simulink library "LIB_Warning"  (R2018b)
settings: Solver=VariableStepAuto  StartTime=0.0  StopTime=10.0  RelTol=1e-3
undefined symbols (not defined in the file or in its folder): eRespiratorStates, eSupervisorStates, rDecWarning, rIncpEndError, rIncpMinError, rIncpPlateauError, tBatteryErrorConfirmationDelay, tTBlowerMotorErrorConfirmationDelay
libraries: simulink x15, simulink_extras x3
settings Model: Creator=BRAUL  LastModifiedBy=BRAUL

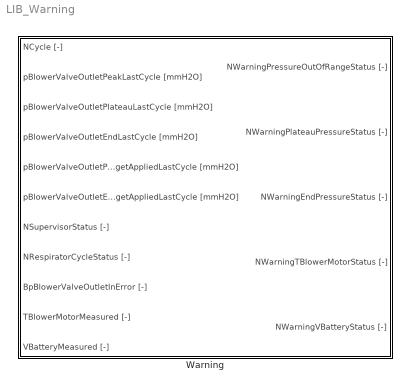
== system LIB_Warning ==
  Warning : Subsystem
      settings: AttributesFormatString=%<ReferenceBlock>

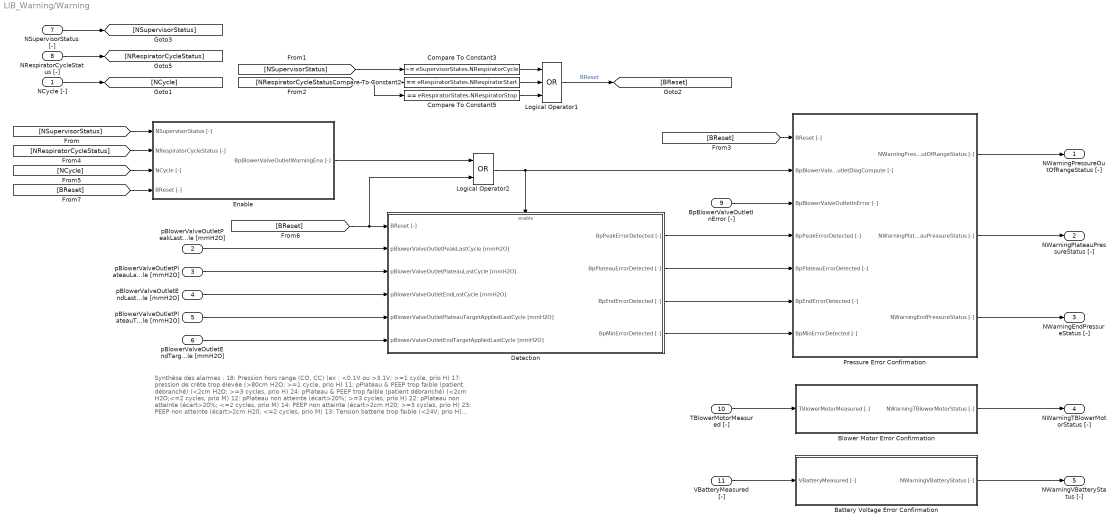
== system LIB_Warning/Warning ==
  note: Synthèse des alarmes :
      |
      | 18: Pression hors range (CO, CC) (ex : <0.1V ou >3.1V; >=1 cycle, prio H)
      | 17: pression de crête trop élevée (>80cm H2O; >=1 cycle, prio H)
      | 11: pPlateau & PEEP trop faible (patient débranché) (<2cm H2O; >=3 cycles, prio H)
      | 24: pPlateau & PEEP trop faible (patient débranché) (<2cm H2O;<=2 cycles, prio M)
      |
      | 12: pPlateau non atteinte (écart>20%; >=3 cycles, prio H)
      | 22: pPlateau non atteinte (écart>20%; <=2 cycles, prio M)
      |
      | 14: PEEP non atteinte (écart>2cm H20; >=3 cycles, prio H)
      | 23: PEEP non atteinte (écart>2cm H20; <=2 cycles, prio M)
      |
      | 13: Tension batterie trop faible (<24V; prio H)
      | 21: Tension batterie faible (<24.6V; prio M)
      | 31: Tension alimentation faible ( <=> secteur débranché)(<27V; prio L)
      |
      | 15: T moteur blower trop élevée (tempé>80°C; prio H)
  NCycle [-] : Inport
  pBlowerValveOutletPeakLastCycle [mmH2O] : Inport  Port=2
  pBlowerValveOutletPlateauLastCycle [mmH2O] : Inport  Port=3
  pBlowerValveOutletEndLastCycle [mmH2O] : Inport  Port=4
  pBlowerValveOutletPlateauTargetAppliedLastCycle [mmH2O] : Inport  Port=5
  pBlowerValveOutletEndTargetAppliedLastCycle [mmH2O] : Inport  Port=6
  NSupervisorStatus [-] : Inport  Port=7
  NRespiratorCycleStatus [-] : Inport  Port=8
  BpBlowerValveOutletInError [-] : Inport  Port=9
  TBlowerMotorMeasured [-] : Inport  Port=10
  VBatteryMeasured [-] : Inport  Port=11
  Battery Voltage Error Confirmation : Subsystem
  Blower Motor Error Confirmation : Subsystem
  Compare To Constant2 : simulink/Logic and Bit Operations/Compare To Constant  relop===  const=eRespiratorStates.NRespiratorStart  OutDataTypeStr=boolean
  Compare To Constant3 : simulink/Logic and Bit Operations/Compare To Constant  relop=~=  const=eSupervisorStates.NRespiratorCycle  OutDataTypeStr=boolean
  Compare To Constant5 : simulink/Logic and Bit Operations/Compare To Constant  relop===  const=eRespiratorStates.NRespiratorStop  OutDataTypeStr=boolean
  Detection : Subsystem
  Enable : Subsystem
  Logical Operator1 : Logic  Operator=OR  Inputs=3  AllPortsSameDT=off  OutDataTypeStr=boolean
  Logical Operator2 : Logic  Operator=OR  AllPortsSameDT=off  OutDataTypeStr=boolean
  Pressure Error Confirmation : Subsystem
  NWarningPressureOutOfRangeStatus [-] : Outport
  NWarningPlateauPressureStatus [-] : Outport  Port=2
  NWarningEndPressureStatus [-] : Outport  Port=3
  NWarningTBlowerMotorStatus [-] : Outport  Port=4
  NWarningVBatteryStatus [-] : Outport  Port=5
  wires:
  pBlowerValveOutletPlateauTargetAppliedLastCycle [mmH2O]/1 -> Detection/5(pBlowerValveOutletPlateauTargetAppliedLastCycle [mmH2O])
  pBlowerValveOutletEndLastCycle [mmH2O]/1 -> Detection/4(pBlowerValveOutletEndLastCycle [mmH2O])
  Battery Voltage Error Confirmation/1(NWarningVBatteryStatus [-]) -> NWarningVBatteryStatus [-]/1
  Blower Motor Error Confirmation/1(NWarningTBlowerMotorStatus [-]) -> NWarningTBlowerMotorStatus [-]/1
  Pressure Error Confirmation/3(NWarningEndPressureStatus [-]) -> NWarningEndPressureStatus [-]/1
  Pressure Error Confirmation/2(NWarningPlateauPressureStatus [-]) -> NWarningPlateauPressureStatus [-]/1
  Pressure Error Confirmation/1(NWarningPressureOutOfRangeStatus [-]) -> NWarningPressureOutOfRangeStatus [-]/1
  Enable/1(BpBlowerValveOutletWarningEna [-]) -> Logical Operator2/1
  [BReset] -> Logical Operator2/2, Detection/1(BReset [-])
  Logical Operator2/1 -> Detection/Enable, Pressure Error Confirmation/2(BpBlowerValveOutletDiagCompute [-])
  BpBlowerValveOutletInError [-]/1 -> Pressure Error Confirmation/3(BpBlowerValveOutletInError [-])
  TBlowerMotorMeasured [-]/1 -> Blower Motor Error Confirmation/1(TBlowerMotorMeasured [-])
  VBatteryMeasured [-]/1 -> Battery Voltage Error Confirmation/1(VBatteryMeasured [-])
  [BReset] -> Enable/4(BReset [-])
  [NCycle] -> Enable/3(NCycle [-])
  [NRespiratorCycleStatus] -> Enable/2(NRespiratorCycleStatus [-])
  pBlowerValveOutletEndTargetAppliedLastCycle [mmH2O]/1 -> Detection/6(pBlowerValveOutletEndTargetAppliedLastCycle [mmH2O])
  pBlowerValveOutletPlateauLastCycle [mmH2O]/1 -> Detection/3(pBlowerValveOutletPlateauLastCycle [mmH2O])
  pBlowerValveOutletPeakLastCycle [mmH2O]/1 -> Detection/2(pBlowerValveOutletPeakLastCycle [mmH2O])
  [BReset] -> Pressure Error Confirmation/1(BReset [-])
  [NSupervisorStatus] -> Enable/1(NSupervisorStatus [-])
  NCycle [-]/1 -> [NCycle]
  NRespiratorCycleStatus [-]/1 -> [NRespiratorCycleStatus]
  NSupervisorStatus [-]/1 -> [NSupervisorStatus]
  [NRespiratorCycleStatus] -> Compare To Constant5/1, Compare To Constant2/1
  Compare To Constant5/1 -> Logical Operator1/3
  [NSupervisorStatus] -> Compare To Constant3/1
  Compare To Constant3/1 -> Logical Operator1/1
  Logical Operator1/1 -> [BReset]  "BReset"
  Compare To Constant2/1 -> Logical Operator1/2
  Detection/4(BpMinErrorDetected [-]) -> Pressure Error Confirmation/7(BpMinErrorDetected [-])
  Detection/3(BpEndErrorDetected [-]) -> Pressure Error Confirmation/6(BpEndErrorDetected [-])
  Detection/2(BpPlateauErrorDetected [-]) -> Pressure Error Confirmation/5(BpPlateauErrorDetected [-])
  Detection/1(BpPeakErrorDetected [-]) -> Pressure Error Confirmation/4(BpPeakErrorDetected [-])

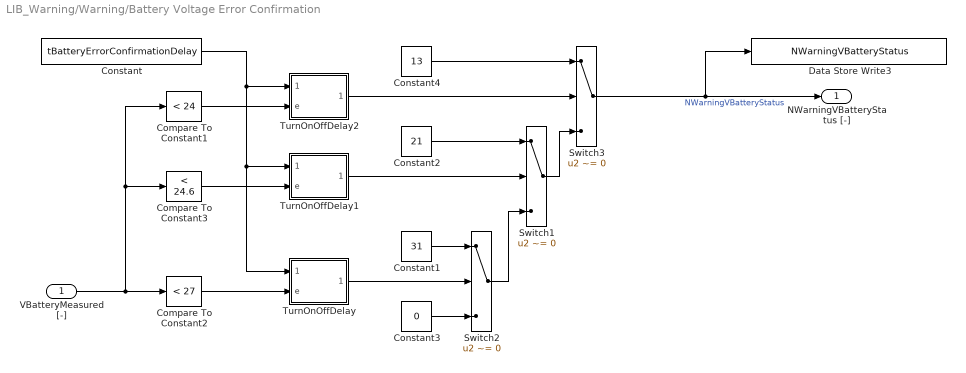
== system LIB_Warning/Warning/Battery Voltage Error Confirmation ==
  VBatteryMeasured [-] : Inport
  Compare To Constant1 : simulink/Logic and Bit Operations/Compare To Constant  relop=<  const=24  OutDataTypeStr=boolean
  Compare To Constant2 : simulink/Logic and Bit Operations/Compare To Constant  relop=<  const=27  OutDataTypeStr=boolean
  Compare To Constant3 : simulink/Logic and Bit Operations/Compare To Constant  relop=<  const=24.6  OutDataTypeStr=boolean
  Constant : Constant  Value=tBatteryErrorConfirmationDelay  OutDataTypeStr=single
  Constant1 : Constant  Value=31  OutDataTypeStr=uint8
  Constant2 : Constant  Value=21  OutDataTypeStr=uint8
  Constant3 : Constant  Value=0  OutDataTypeStr=uint8
  Constant4 : Constant  Value=13  OutDataTypeStr=uint8
  Data Store Write3 : DataStoreWrite  DataStoreName=NWarningVBatteryStatus
  Switch1 : Switch  Criteria=u2 ~= 0
      settings: AttributesFormatString=%<Criteria>
  Switch2 : Switch  Criteria=u2 ~= 0
      settings: AttributesFormatString=%<Criteria>
  Switch3 : Switch  Criteria=u2 ~= 0
      settings: AttributesFormatString=%<Criteria>
  TurnOnOffDelay : Subsystem  mask(TurnOn/OffDelay){DelayType=Turn On Delay, OutDataType=boolean}
      mask prompts: DelayType "Delay Type"; OutDataType "Out Data Type"
      mask help: Bloc de confirmation de montée/chute si e est/n'est plus vrai pendant une durée T (en secondes)
      mask init:
      | LogicBlocks=find_system(gcbh,'LookUnderMasks','all','FollowLinks','On','SearchDepth','1','BlockType','Logic');
      | DetectionBlock=find_system(gcbh,'LookUnderMasks','all','FollowLinks','On','SearchDepth','1','MaskType','DETECTIONFRONT');
      | if DelayType==1
      | set_param(LogicBlocks(1),'Operator','AND');
      | set_param(LogicBlocks(2),'Operator','AND');
      | set_param(DetectionBlock,'FrontType','Rising');
      | FrontIconY=[0.2 0.2 0.6 0.6];
      | else
      | set_param(LogicBlocks(1),'Operator','OR')
      | set_param(LogicBlocks(2),'Operator','NOT');
      | set_param(DetectionBlock,'FrontType','Falling');
      | FrontIconY=[0.6 0.6 0.2 0.2];
      | end
      | 
      | ConversionBlock=find_system(gcbh,'LookUnderMasks','all','FollowLinks','On','SearchDepth','1','BlockType','DataTypeConversion');
      | DataTypeOptionsStr=[{'Inherit: Inherit via back propagation'},{'double'},{'single'},{'int8'},{'uint8'},{'int16'},{'uint16'},{'int32'},{'uint32'},{'boolean'},{'fixdt(1,16)'},{'fixdt(1,16,0)'},{'fixdt(1,16,2^0,0)'},{'Enum: <class name>'},{'<data type expression>'}]
      | set_param(ConversionBlock,'OutDataTypeStr',DataTypeOptionsStr{OutDataType});
      settings: AttributesFormatString=%<StaticLinkStatus>
      mask TypeOptions DelayType: Turn On Delay | Turn Off Delay
      mask TypeOptions OutDataType: Inherit: Inherit via back propagation | double | single | int8 | uint8 | int16 | uint16 | int32 | uint32 | boolean | fixdt(1,16) | fixdt(1,16,0) | fixdt(1,16,2^0,0) | Enum: <class name> | <data type expression>
      mask Display:
      | plot([0.3 0.6 0.6 0.9], FrontIconY);
      | port_label('input',1,'T [s]')
      | port_label('input',2,'e')
      | text(0.4,0.4, 'T');
  TurnOnOffDelay1 : Subsystem  mask(TurnOn/OffDelay){DelayType=Turn On Delay, OutDataType=boolean}
      mask prompts: DelayType "Delay Type"; OutDataType "Out Data Type"
      mask help: Bloc de confirmation de montée/chute si e est/n'est plus vrai pendant une durée T (en secondes)
      mask init: same as LIB_Warning/Warning/Battery Voltage Error Confirmation/TurnOnOffDelay
      settings: AttributesFormatString=%<StaticLinkStatus>
      mask TypeOptions DelayType: Turn On Delay | Turn Off Delay
      mask TypeOptions OutDataType: Inherit: Inherit via back propagation | double | single | int8 | uint8 | int16 | uint16 | int32 | uint32 | boolean | fixdt(1,16) | fixdt(1,16,0) | fixdt(1,16,2^0,0) | Enum: <class name> | <data type expression>
      mask Display:
      | plot([0.3 0.6 0.6 0.9], FrontIconY);
      | port_label('input',1,'T [s]')
      | port_label('input',2,'e')
      | text(0.4,0.4, 'T');
  TurnOnOffDelay2 : Subsystem  mask(TurnOn/OffDelay){DelayType=Turn On Delay, OutDataType=boolean}
      mask prompts: DelayType "Delay Type"; OutDataType "Out Data Type"
      mask help: Bloc de confirmation de montée/chute si e est/n'est plus vrai pendant une durée T (en secondes)
      mask init: same as LIB_Warning/Warning/Battery Voltage Error Confirmation/TurnOnOffDelay
      settings: AttributesFormatString=%<StaticLinkStatus>
      mask TypeOptions DelayType: Turn On Delay | Turn Off Delay
      mask TypeOptions OutDataType: Inherit: Inherit via back propagation | double | single | int8 | uint8 | int16 | uint16 | int32 | uint32 | boolean | fixdt(1,16) | fixdt(1,16,0) | fixdt(1,16,2^0,0) | Enum: <class name> | <data type expression>
      mask Display:
      | plot([0.3 0.6 0.6 0.9], FrontIconY);
      | port_label('input',1,'T [s]')
      | port_label('input',2,'e')
      | text(0.4,0.4, 'T');
  NWarningVBatteryStatus [-] : Outport
  wires:
  Constant/1 -> TurnOnOffDelay2/1(DelayTime), TurnOnOffDelay1/1(DelayTime), TurnOnOffDelay/1(DelayTime)
  TurnOnOffDelay/1(Timer_end) -> Switch2/2
  TurnOnOffDelay1/1(Timer_end) -> Switch1/2
  TurnOnOffDelay2/1(Timer_end) -> Switch3/2
  Compare To Constant3/1 -> TurnOnOffDelay1/2(e)
  Compare To Constant1/1 -> TurnOnOffDelay2/2(e)
  Compare To Constant2/1 -> TurnOnOffDelay/2(e)
  Constant4/1 -> Switch3/1
  Constant2/1 -> Switch1/1
  Constant1/1 -> Switch2/1
  Constant3/1 -> Switch2/3
  Switch3/1 -> NWarningVBatteryStatus [-]/1, Data Store Write3/1  "NWarningVBatteryStatus"
  Switch1/1 -> Switch3/3
  Switch2/1 -> Switch1/3
  VBatteryMeasured [-]/1 -> Compare To Constant3/1, Compare To Constant1/1, Compare To Constant2/1

== system LIB_Warning/Warning/Blower Motor Error Confirmation ==
  TBlowerMotorMeasured [-] : Inport
  Compare To Constant2 : simulink/Logic and Bit Operations/Compare To Constant  relop=>  const=80  OutDataTypeStr=boolean
  Constant : Constant  Value=tTBlowerMotorErrorConfirmationDelay  OutDataTypeStr=single
  Constant1 : Constant  Value=15  OutDataTypeStr=uint8
  Constant3 : Constant  Value=0  OutDataTypeStr=uint8
  Data Store Write3 : DataStoreWrite  DataStoreName=NWarningTBlowerMotorStatus
  Switch2 : Switch  Criteria=u2 ~= 0
      settings: AttributesFormatString=%<Criteria>
  TurnOnOffDelay : Subsystem  mask(TurnOn/OffDelay){DelayType=Turn On Delay, OutDataType=boolean}
      mask prompts: DelayType "Delay Type"; OutDataType "Out Data Type"
      mask help: Bloc de confirmation de montée/chute si e est/n'est plus vrai pendant une durée T (en secondes)
      mask init: same as LIB_Warning/Warning/Battery Voltage Error Confirmation/TurnOnOffDelay
      settings: AttributesFormatString=%<StaticLinkStatus>
      mask TypeOptions DelayType: Turn On Delay | Turn Off Delay
      mask TypeOptions OutDataType: Inherit: Inherit via back propagation | double | single | int8 | uint8 | int16 | uint16 | int32 | uint32 | boolean | fixdt(1,16) | fixdt(1,16,0) | fixdt(1,16,2^0,0) | Enum: <class name> | <data type expression>
      mask Display:
      | plot([0.3 0.6 0.6 0.9], FrontIconY);
      | port_label('input',1,'T [s]')
      | port_label('input',2,'e')
      | text(0.4,0.4, 'T');
  NWarningTBlowerMotorStatus [-] : Outport
  wires:
  TBlowerMotorMeasured [-]/1 -> Compare To Constant2/1
  Switch2/1 -> NWarningTBlowerMotorStatus [-]/1, Data Store Write3/1  "NWarningTBlowerMotorStatus"
  Constant3/1 -> Switch2/3
  Constant1/1 -> Switch2/1
  Compare To Constant2/1 -> TurnOnOffDelay/2(e)
  TurnOnOffDelay/1(Timer_end) -> Switch2/2
  Constant/1 -> TurnOnOffDelay/1(DelayTime)

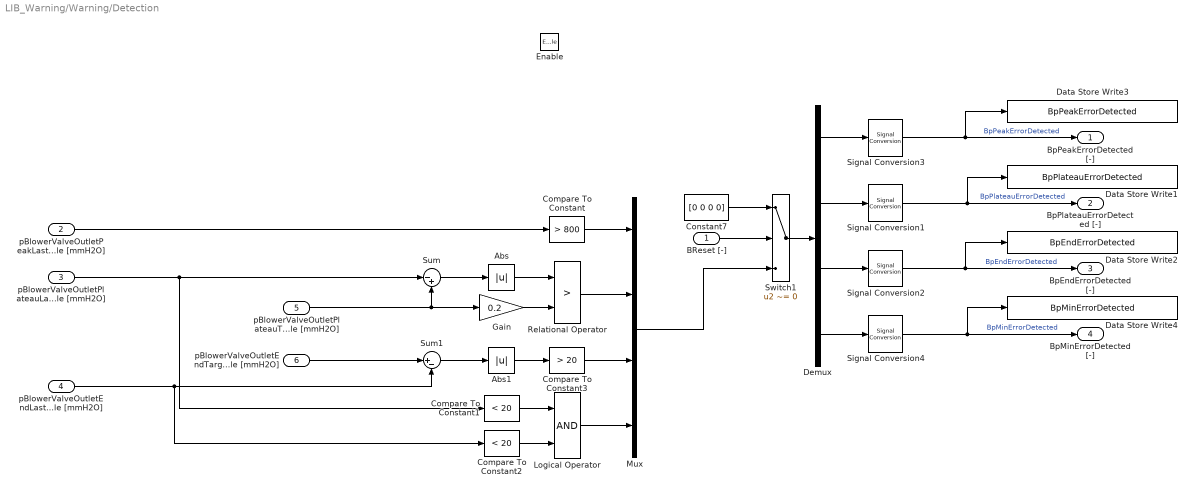
== system LIB_Warning/Warning/Detection ==
  BReset [-] : Inport
  pBlowerValveOutletPeakLastCycle [mmH2O] : Inport  Port=2
  pBlowerValveOutletPlateauLastCycle [mmH2O] : Inport  Port=3
  pBlowerValveOutletEndLastCycle [mmH2O] : Inport  Port=4
  pBlowerValveOutletPlateauTargetAppliedLastCycle [mmH2O] : Inport  Port=5
  pBlowerValveOutletEndTargetAppliedLastCycle [mmH2O] : Inport  Port=6
  Enable : EnablePort
  Abs : Abs
  Abs1 : Abs
  Compare To Constant : simulink/Logic and Bit Operations/Compare To Constant  relop=>  const=800  OutDataTypeStr=boolean
  Compare To Constant1 : simulink/Logic and Bit Operations/Compare To Constant  relop=<  const=20  OutDataTypeStr=boolean
  Compare To Constant2 : simulink/Logic and Bit Operations/Compare To Constant  relop=<  const=20  OutDataTypeStr=boolean
  Compare To Constant3 : simulink/Logic and Bit Operations/Compare To Constant  relop=>  const=20  OutDataTypeStr=boolean
  Constant7 : Constant  Value=[0 0 0 0]  OutDataTypeStr=boolean
  Data Store Write1 : DataStoreWrite  DataStoreName=BpPlateauErrorDetected
  Data Store Write2 : DataStoreWrite  DataStoreName=BpEndErrorDetected
  Data Store Write3 : DataStoreWrite  DataStoreName=BpPeakErrorDetected
  Data Store Write4 : DataStoreWrite  DataStoreName=BpMinErrorDetected
  Demux : Demux
  Gain : Gain  Gain=0.2
  Logical Operator : Logic  AllPortsSameDT=off  OutDataTypeStr=boolean
  Mux : Mux
  Relational Operator : RelationalOperator  Operator=>  OutDataTypeStr=boolean  RndMeth=Simplest
  Signal Conversion{1..4} (4 alike) : SignalConversion  OverrideOpt=off
  Sum : Sum  Inputs=|-+
  Sum1 : Sum  Inputs=|+-
  Switch1 : Switch  Criteria=u2 ~= 0
      settings: AttributesFormatString=%<Criteria>
  BpPeakErrorDetected [-] : Outport
  BpPlateauErrorDetected [-] : Outport  Port=2
  BpEndErrorDetected [-] : Outport  Port=3
  BpMinErrorDetected [-] : Outport  Port=4
  wires:
  Signal Conversion4/1 -> BpMinErrorDetected [-]/1, Data Store Write4/1  "BpMinErrorDetected"
  Signal Conversion2/1 -> BpEndErrorDetected [-]/1, Data Store Write2/1  "BpEndErrorDetected"
  Signal Conversion1/1 -> BpPlateauErrorDetected [-]/1, Data Store Write1/1  "BpPlateauErrorDetected"
  Signal Conversion3/1 -> BpPeakErrorDetected [-]/1, Data Store Write3/1  "BpPeakErrorDetected"
  Demux/4 -> Signal Conversion4/1
  Demux/3 -> Signal Conversion2/1
  Demux/2 -> Signal Conversion1/1
  Demux/1 -> Signal Conversion3/1
  Logical Operator/1 -> Mux/4
  Compare To Constant3/1 -> Mux/3
  Relational Operator/1 -> Mux/2
  Compare To Constant/1 -> Mux/1
  Mux/1 -> Switch1/3
  Switch1/1 -> Demux/1
  BReset [-]/1 -> Switch1/2
  Constant7/1 -> Switch1/1
  Abs1/1 -> Compare To Constant3/1
  Abs/1 -> Relational Operator/1
  Gain/1 -> Relational Operator/2
  pBlowerValveOutletPlateauTargetAppliedLastCycle [mmH2O]/1 -> Sum/2, Gain/1
  Compare To Constant1/1 -> Logical Operator/1
  Compare To Constant2/1 -> Logical Operator/2
  pBlowerValveOutletEndLastCycle [mmH2O]/1 -> Sum1/2, Compare To Constant2/1
  pBlowerValveOutletEndTargetAppliedLastCycle [mmH2O]/1 -> Sum1/1
  Sum1/1 -> Abs1/1
  pBlowerValveOutletPlateauLastCycle [mmH2O]/1 -> Compare To Constant1/1, Sum/1
  Sum/1 -> Abs/1
  pBlowerValveOutletPeakLastCycle [mmH2O]/1 -> Compare To Constant/1

== system LIB_Warning/Warning/Enable ==
  NSupervisorStatus [-] : Inport
  NRespiratorCycleStatus [-] : Inport  Port=2
  NCycle [-] : Inport  Port=3
  BReset [-] : Inport  Port=4
  Compare To Constant : simulink/Logic and Bit Operations/Compare To Constant  relop=>  const=1  OutDataTypeStr=boolean
  Compare To Constant1 : simulink/Logic and Bit Operations/Compare To Constant  relop===  const=eRespiratorStates.NRespiratorInInhalationPhase1  OutDataTypeStr=boolean
  Compare To Constant4 : simulink/Logic and Bit Operations/Compare To Constant  relop===  const=eSupervisorStates.NRespiratorCycle  OutDataTypeStr=boolean
  Constant6 : Constant  OutDataTypeStr=boolean
  Constant7 : Constant  Value=0  OutDataTypeStr=boolean
  Data Store Write3 : DataStoreWrite  DataStoreName=BpBlowerValveOutletWarningEna
  Detect Increase : simulink/Logic and Bit Operations/Detect Increase  vinit=0.0  OutDataTypeStr=boolean
  Logical Operator2 : Logic  Inputs=3  AllPortsSameDT=off  OutDataTypeStr=boolean
  Switch1 : Switch  Criteria=u2 ~= 0
      settings: AttributesFormatString=%<Criteria>
  Switch4 : Switch  Criteria=u2 ~= 0
      settings: AttributesFormatString=%<Criteria>
  Unit Delay1 : UnitDelay  SampleTime=-1
      settings: AttributesFormatString=%<InitialCondition>
  BpBlowerValveOutletWarningEna [-] : Outport
  wires:
  Compare To Constant/1 -> Switch4/2
  BReset [-]/1 -> Switch1/2
  NSupervisorStatus [-]/1 -> Compare To Constant4/1
  Detect Increase/1 -> Logical Operator2/2
  Constant7/1 -> Switch1/1
  NCycle [-]/1 -> Compare To Constant/1
  Unit Delay1/1 -> Switch4/3
  Switch1/1 -> Unit Delay1/1, Logical Operator2/3
  Constant6/1 -> Switch4/1
  NRespiratorCycleStatus [-]/1 -> Compare To Constant1/1
  Switch4/1 -> Switch1/3
  Logical Operator2/1 -> BpBlowerValveOutletWarningEna [-]/1, Data Store Write3/1  "BpBlowerValveOutletWarningEna"
  Compare To Constant1/1 -> Detect Increase/1
  Compare To Constant4/1 -> Logical Operator2/1

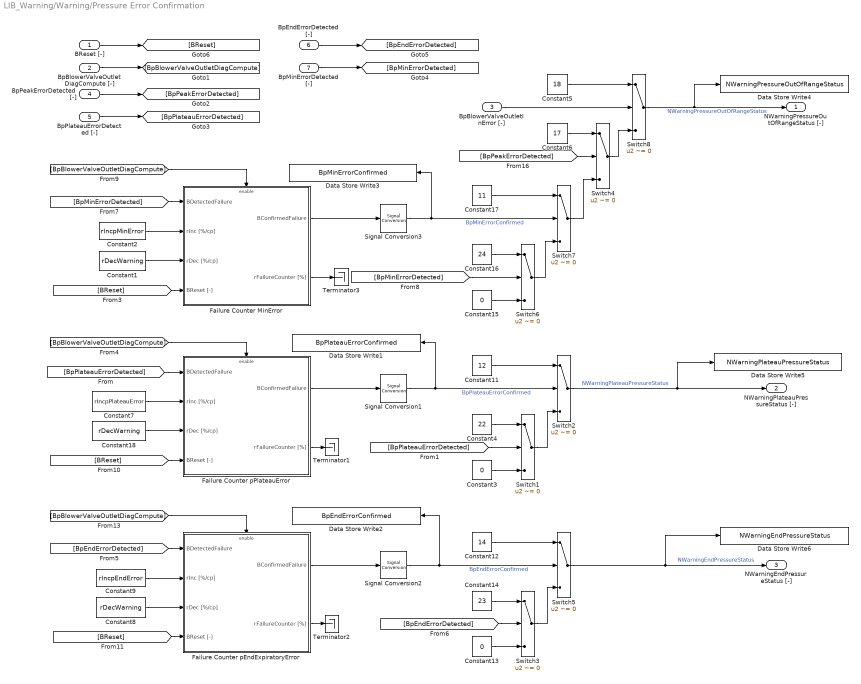
== system LIB_Warning/Warning/Pressure Error Confirmation ==
  BReset [-] : Inport
  BpBlowerValveOutletDiagCompute [-] : Inport  Port=2
  BpBlowerValveOutletInError [-] : Inport  Port=3
  BpPeakErrorDetected [-] : Inport  Port=4
  BpPlateauErrorDetected [-] : Inport  Port=5
  BpEndErrorDetected [-] : Inport  Port=6
  BpMinErrorDetected [-] : Inport  Port=7
  Constant1 : Constant  Value=rDecWarning  OutDataTypeStr=single
  Constant11 : Constant  Value=12  OutDataTypeStr=uint8
  Constant12 : Constant  Value=14  OutDataTypeStr=uint8
  Constant13 : Constant  Value=0  OutDataTypeStr=uint8
  Constant14 : Constant  Value=23  OutDataTypeStr=uint8
  Constant15 : Constant  Value=0  OutDataTypeStr=uint8
  Constant16 : Constant  Value=24  OutDataTypeStr=uint8
  Constant17 : Constant  Value=11  OutDataTypeStr=uint8
  Constant18 : Constant  Value=rDecWarning  OutDataTypeStr=single
  Constant2 : Constant  Value=rIncpMinError  OutDataTypeStr=single
  Constant3 : Constant  Value=0  OutDataTypeStr=uint8
  Constant4 : Constant  Value=22  OutDataTypeStr=uint8
  Constant5 : Constant  Value=18  OutDataTypeStr=uint8
  Constant6 : Constant  Value=17  OutDataTypeStr=uint8
  Constant7 : Constant  Value=rIncpPlateauError  OutDataTypeStr=single
  Constant8 : Constant  Value=rDecWarning  OutDataTypeStr=single
  Constant9 : Constant  Value=rIncpEndError  OutDataTypeStr=single
  Data Store Write1 : DataStoreWrite  DataStoreName=BpPlateauErrorConfirmed
  Data Store Write2 : DataStoreWrite  DataStoreName=BpEndErrorConfirmed
  Data Store Write3 : DataStoreWrite  DataStoreName=BpMinErrorConfirmed
  Data Store Write4 : DataStoreWrite  DataStoreName=NWarningPressureOutOfRangeStatus
  Data Store Write5 : DataStoreWrite  DataStoreName=NWarningPlateauPressureStatus
  Data Store Write6 : DataStoreWrite  DataStoreName=NWarningEndPressureStatus
  Failure Counter MinError : Subsystem  TreatAsAtomicUnit=on  mask(Failure Counter){temp=off, TSample=10, ena=on}
      mask prompts: temp "Is Temporal?"; TSample "Sample Time (ms)"; ena "Need to be Enable?"
      mask init:
      | %Find inputs to change name
      | rInc=find_system(gcbh,'LookUnderMasks','all','FollowLinks','on','RegExp','on','Name','rInc');
      | rDec=find_system(gcbh,'LookUnderMasks','all','FollowLinks','on','RegExp','on','Name','rDec');
      | rFail=find_system(gcbh,'LookUnderMasks','all','FollowLinks','on','RegExp','on','Name','rFail');
      | % Active enable
      | ena_block=find_system(gcbh,'LookUnderMasks','all','FollowLinks','on','Name','enable');
      | if ena && isempty(ena_block)  
      |     add_block('simulink/Ports & Subsystems/Enable',[gcb,'/enable'])
      | elseif not(ena) && not(isempty(ena_block))
      |     delete_block([gcb,'/enable']);
      | end
      | 
      | %Verify if Temporal or not
      | if temp
      |     set_param([gcb '/Sample'],'Value',mat2str(eval(TSample)))
      |     %sample=replace_block(gcbh,'Name','Sample','GDElib_functions/SampleTime','noprompt');
      |     %set_param(gcb,'DataType','single','TSample',mat2str(eval(TSample)/1000));
      |     set_param(rInc,'Name','rInc [%/ms]')
      |     set_param(rDec,'Name','rDec [%/ms]')
      |     set_param(rFail,'Name','rFailureCounter [%]')
      |     status=['Temporal \n' TSample ' ms'];
      | else
      |     set_param([gcb,'/Sample'],'Value','1');
      |     set_param(rInc,'Name','rInc [%/cp]')
      |     set_param(rDec,'Name','rDec [%/cp]')
      |     set_param(rFail,'Name','rFailureCounter [%]')
      |     status='Not Temporal';
      |     
      | end
      settings: AttributesFormatString=%<StaticLinkStatus>
      mask Callback temp:
      | maskedit_FailC=get_param(gcb,'temp');
      | vis_FailC = get_param(gcb, 'maskvisibilities');
      | vis_FailC{2} = maskedit_FailC;
      | set_param(gcb,'maskvisibilities',vis_FailC);
      | clear vis_FailC maskedit_FailC;
      mask TypeOptions TSample: 1 | 2 | 5 | 10 | 20 | 50 | 100 | 1000
      mask Display: disp(status)
  Failure Counter pEndExpiratoryError : Subsystem  TreatAsAtomicUnit=on  mask(Failure Counter){temp=off, TSample=10, ena=on}
      mask prompts: temp "Is Temporal?"; TSample "Sample Time (ms)"; ena "Need to be Enable?"
      mask init: same as LIB_Warning/Warning/Pressure Error Confirmation/Failure Counter MinError
      settings: AttributesFormatString=%<StaticLinkStatus>
      mask Callback temp:
      | maskedit_FailC=get_param(gcb,'temp');
      | vis_FailC = get_param(gcb, 'maskvisibilities');
      | vis_FailC{2} = maskedit_FailC;
      | set_param(gcb,'maskvisibilities',vis_FailC);
      | clear vis_FailC maskedit_FailC;
      mask TypeOptions TSample: 1 | 2 | 5 | 10 | 20 | 50 | 100 | 1000
      mask Display: disp(status)
  Failure Counter pPlateauError : Subsystem  TreatAsAtomicUnit=on  mask(Failure Counter){temp=off, TSample=10, ena=on}
      mask prompts: temp "Is Temporal?"; TSample "Sample Time (ms)"; ena "Need to be Enable?"
      mask init: same as LIB_Warning/Warning/Pressure Error Confirmation/Failure Counter MinError
      settings: AttributesFormatString=%<StaticLinkStatus>
      mask Callback temp:
      | maskedit_FailC=get_param(gcb,'temp');
      | vis_FailC = get_param(gcb, 'maskvisibilities');
      | vis_FailC{2} = maskedit_FailC;
      | set_param(gcb,'maskvisibilities',vis_FailC);
      | clear vis_FailC maskedit_FailC;
      mask TypeOptions TSample: 1 | 2 | 5 | 10 | 20 | 50 | 100 | 1000
      mask Display: disp(status)
  Signal Conversion1 : SignalConversion  OverrideOpt=off
  Signal Conversion2 : SignalConversion  OverrideOpt=off
  Signal Conversion3 : SignalConversion  OverrideOpt=off
  Switch{1..8} (8 alike) : Switch  Criteria=u2 ~= 0
      settings: AttributesFormatString=%<Criteria>
  Terminator1 : Terminator
  Terminator2 : Terminator
  Terminator3 : Terminator
  NWarningPressureOutOfRangeStatus [-] : Outport
  NWarningPlateauPressureStatus [-] : Outport  Port=2
  NWarningEndPressureStatus [-] : Outport  Port=3
  wires:
  [BpPeakErrorDetected] -> Switch4/2
  Constant5/1 -> Switch8/1
  BpBlowerValveOutletInError [-]/1 -> Switch8/2
  Switch4/1 -> Switch8/3
  Switch8/1 -> NWarningPressureOutOfRangeStatus [-]/1, Data Store Write4/1  "NWarningPressureOutOfRangeStatus"
  [BReset] -> Failure Counter pPlateauError/4(BReset [-])
  [BReset] -> Failure Counter pEndExpiratoryError/4(BReset [-])
  [BpBlowerValveOutletDiagCompute] -> Failure Counter pPlateauError/Enable
  [BpBlowerValveOutletDiagCompute] -> Failure Counter MinError/Enable
  [BReset] -> Failure Counter MinError/4(BReset [-])
  BReset [-]/1 -> [BReset]
  Switch5/1 -> NWarningEndPressureStatus [-]/1, Data Store Write6/1  "NWarningEndPressureStatus"
  Switch2/1 -> NWarningPlateauPressureStatus [-]/1, Data Store Write5/1  "NWarningPlateauPressureStatus"
  Switch7/1 -> Switch4/3
  Constant17/1 -> Switch7/1
  Constant16/1 -> Switch6/1
  Switch6/1 -> Switch7/3
  Signal Conversion3/1 -> Switch7/2, Data Store Write3/1  "BpMinErrorConfirmed"
  Failure Counter MinError/1(BConfirmedFailure) -> Signal Conversion3/1
  Failure Counter MinError/2(rFailureCounter [%]) -> Terminator3/1
  Constant15/1 -> Switch6/3
  [BpMinErrorDetected] -> Switch6/2
  [BpMinErrorDetected] -> Failure Counter MinError/1(BDetectedFailure)
  Failure Counter pEndExpiratoryError/2(rFailureCounter [%]) -> Terminator2/1
  Constant14/1 -> Switch3/1
  [BpEndErrorDetected] -> Switch3/2
  Switch3/1 -> Switch5/3
  Constant13/1 -> Switch3/3
  Constant12/1 -> Switch5/1
  Signal Conversion2/1 -> Switch5/2, Data Store Write2/1  "BpEndErrorConfirmed"
  Failure Counter pEndExpiratoryError/1(BConfirmedFailure) -> Signal Conversion2/1
  [BpEndErrorDetected] -> Failure Counter pEndExpiratoryError/1(BDetectedFailure)
  Constant11/1 -> Switch2/1
  Switch1/1 -> Switch2/3
  Constant4/1 -> Switch1/1
  [BpPlateauErrorDetected] -> Switch1/2
  Constant3/1 -> Switch1/3
  [BpPlateauErrorDetected] -> Failure Counter pPlateauError/1(BDetectedFailure)
  Constant6/1 -> Switch4/1
  BpEndErrorDetected [-]/1 -> [BpEndErrorDetected]
  BpMinErrorDetected [-]/1 -> [BpMinErrorDetected]
  BpPlateauErrorDetected [-]/1 -> [BpPlateauErrorDetected]
  BpPeakErrorDetected [-]/1 -> [BpPeakErrorDetected]
  Failure Counter pPlateauError/2(rFailureCounter [%]) -> Terminator1/1
  Failure Counter pPlateauError/1(BConfirmedFailure) -> Signal Conversion1/1
  Signal Conversion1/1 -> Switch2/2, Data Store Write1/1  "BpPlateauErrorConfirmed"
  Constant1/1 -> Failure Counter MinError/3(rDec [%/cp])
  Constant2/1 -> Failure Counter MinError/2(rInc [%/cp])
  [BpBlowerValveOutletDiagCompute] -> Failure Counter pEndExpiratoryError/Enable
  Constant8/1 -> Failure Counter pEndExpiratoryError/3(rDec [%/cp])
  Constant9/1 -> Failure Counter pEndExpiratoryError/2(rInc [%/cp])
  Constant18/1 -> Failure Counter pPlateauError/3(rDec [%/cp])
  Constant7/1 -> Failure Counter pPlateauError/2(rInc [%/cp])
  BpBlowerValveOutletDiagCompute [-]/1 -> [BpBlowerValveOutletDiagCompute]

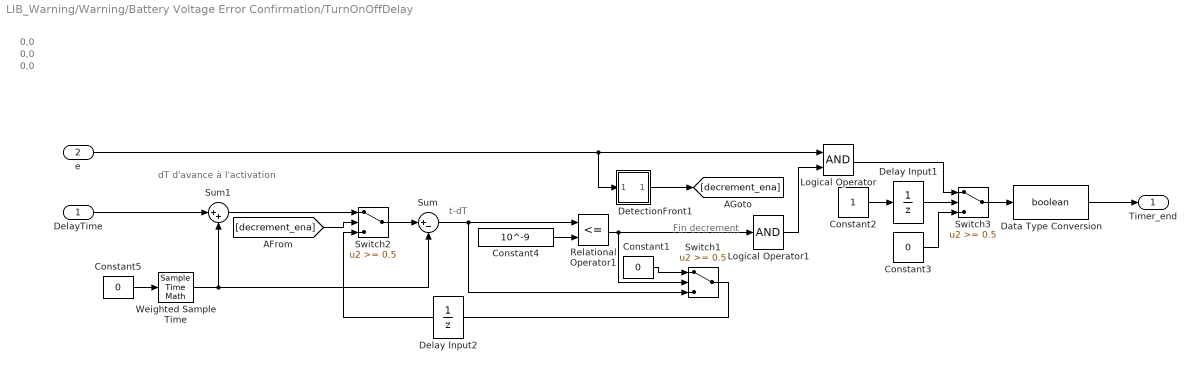
== system LIB_Warning/Warning/Battery Voltage Error Confirmation/TurnOnOffDelay ==
  note: dT d'avance à l'activation
  note: t-dT
  note: Fin decrement
  note: 0,0
  note: 0,0
  note: 0,0
  note: 0,0
  note: 0,0
  note: 0,0
  note: 0,0
  DelayTime : Inport
  e : Inport  Port=2
  Constant1 : Constant  Value=0
  Constant2 : Constant
  Constant3 : Constant  Value=0
  Constant4 : Constant  Tag=AM,Constant,0,1,Value;CMP,Value;  Value=10^-9
  Constant5 : Constant  Value=0  SampleTime=-1
  Data Type Conversion : DataTypeConversion  OutDataTypeStr=boolean
  Delay Input1 : UnitDelay  Description=\nStore in Global RAM  SampleTime=-1
  Delay Input2 : UnitDelay  Description=\nStore in Global RAM  SampleTime=-1
  DetectionFront1 : Subsystem  mask(DETECTIONFRONT){FrontType=Rising, InitialValue=0}
      mask prompts: FrontType "Type de front :"; InitialValue "Condition initiale :"
      mask help:
      | Detecte un front sur un signal binaire :
      | - descendant (Falling)
      | - montant (Rising)
      | - les deux (Either).
      mask init:
      | if (FrontType==1);x=[0 1 1 2];y=[0 0 1 1];
      | elseif (FrontType==2);x=[0 1 1 2];y=[1 1 0 0];
      | else;x=[0 1 1 2;3 4 4 5]';y=[0 0 1 1;1 1 0 0]';end;
      mask TypeOptions FrontType: Rising | Falling | Either
      mask Display: plot(x,y)
  Logical Operator : Logic  AllPortsSameDT=off  OutDataTypeStr=boolean
  Logical Operator1 : Logic  Inputs=1  AllPortsSameDT=off  OutDataTypeStr=boolean
  Relational Operator1 : RelationalOperator  Operator=<=  ZeroCross=off  RndMeth=Nearest
  Sum : Sum  Inputs=|+-
  Sum1 : Sum  Inputs=|++
  Switch1 : Switch  Tag=GEN,Threshold;AM,Switch,2,1;CMP,Threshold;  Threshold=0.5  SaturateOnIntegerOverflow=on
  Switch2 : Switch  Tag=GEN,Threshold;AM,Switch,2,1;CMP,Threshold;  Threshold=0.5  SaturateOnIntegerOverflow=on
  Switch3 : Switch  Tag=GEN,Threshold;AM,Switch,2,1;CMP,Threshold;  Threshold=0.5  SaturateOnIntegerOverflow=on
  Weighted Sample Time : SampleTimeMath  TsampMathOp=Ts Only
  Timer_end : Outport
  wires:
  Logical Operator1/1 -> Logical Operator/2
  Constant5/1 -> Weighted Sample Time/1
  e/1 -> Logical Operator/1, DetectionFront1/1(Entree)
  Weighted Sample Time/1 -> Sum1/2, Sum/2
  DelayTime/1 -> Sum1/1
  Sum/1 -> Relational Operator1/1, Switch1/3
  Relational Operator1/1 -> Logical Operator1/1, Switch1/2
  [decrement_ena] -> Switch2/2
  Sum1/1 -> Switch2/1
  Switch2/1 -> Sum/1
  Delay Input2/1 -> Switch2/3
  Constant1/1 -> Switch1/1
  Switch1/1 -> Delay Input2/1
  DetectionFront1/1(Front) -> [decrement_ena]
  Constant4/1 -> Relational Operator1/2
  Constant2/1 -> Delay Input1/1
  Delay Input1/1 -> Switch3/2
  Switch3/1 -> Data Type Conversion/1
  Logical Operator/1 -> Switch3/1
  Constant3/1 -> Switch3/3
  Data Type Conversion/1 -> Timer_end/1

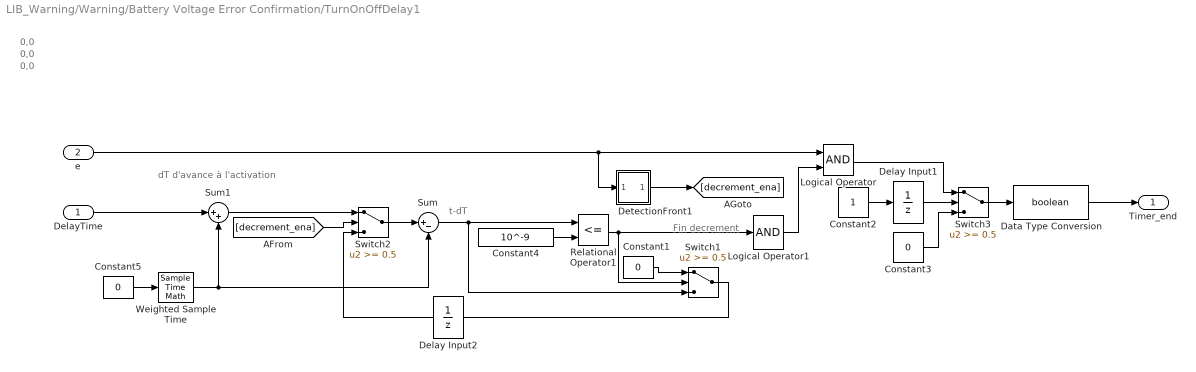
== system LIB_Warning/Warning/Battery Voltage Error Confirmation/TurnOnOffDelay1 ==
  note: 0,0
  note: 0,0
  note: 0,0
  note: 0,0
  note: 0,0
  note: 0,0
  note: 0,0
  note: Fin decrement
  note: t-dT
  note: dT d'avance à l'activation
  DelayTime : Inport
  e : Inport  Port=2
  Constant1 : Constant  Value=0
  Constant2 : Constant
  Constant3 : Constant  Value=0
  Constant4 : Constant  Tag=AM,Constant,0,1,Value;CMP,Value;  Value=10^-9
  Constant5 : Constant  Value=0  SampleTime=-1
  Data Type Conversion : DataTypeConversion  OutDataTypeStr=boolean
  Delay Input1 : UnitDelay  Description=\nStore in Global RAM  SampleTime=-1
  Delay Input2 : UnitDelay  Description=\nStore in Global RAM  SampleTime=-1
  DetectionFront1 : Subsystem  mask(DETECTIONFRONT){FrontType=Rising, InitialValue=0}
      mask prompts: FrontType "Type de front :"; InitialValue "Condition initiale :"
      mask help:
      | Detecte un front sur un signal binaire :
      | - descendant (Falling)
      | - montant (Rising)
      | - les deux (Either).
      mask init:
      | if (FrontType==1);x=[0 1 1 2];y=[0 0 1 1];
      | elseif (FrontType==2);x=[0 1 1 2];y=[1 1 0 0];
      | else;x=[0 1 1 2;3 4 4 5]';y=[0 0 1 1;1 1 0 0]';end;
      mask TypeOptions FrontType: Rising | Falling | Either
      mask Display: plot(x,y)
  Logical Operator : Logic  AllPortsSameDT=off  OutDataTypeStr=boolean
  Logical Operator1 : Logic  Inputs=1  AllPortsSameDT=off  OutDataTypeStr=boolean
  Relational Operator1 : RelationalOperator  Operator=<=  ZeroCross=off  RndMeth=Nearest
  Sum : Sum  Inputs=|+-
  Sum1 : Sum  Inputs=|++
  Switch1 : Switch  Tag=GEN,Threshold;AM,Switch,2,1;CMP,Threshold;  Threshold=0.5  SaturateOnIntegerOverflow=on
  Switch2 : Switch  Tag=GEN,Threshold;AM,Switch,2,1;CMP,Threshold;  Threshold=0.5  SaturateOnIntegerOverflow=on
  Switch3 : Switch  Tag=GEN,Threshold;AM,Switch,2,1;CMP,Threshold;  Threshold=0.5  SaturateOnIntegerOverflow=on
  Weighted Sample Time : SampleTimeMath  TsampMathOp=Ts Only
  Timer_end : Outport
  wires:
  Data Type Conversion/1 -> Timer_end/1
  Constant3/1 -> Switch3/3
  Logical Operator/1 -> Switch3/1
  Switch3/1 -> Data Type Conversion/1
  Delay Input1/1 -> Switch3/2
  Constant2/1 -> Delay Input1/1
  Constant4/1 -> Relational Operator1/2
  DetectionFront1/1(Front) -> [decrement_ena]
  Switch1/1 -> Delay Input2/1
  Constant1/1 -> Switch1/1
  Delay Input2/1 -> Switch2/3
  Switch2/1 -> Sum/1
  Sum1/1 -> Switch2/1
  [decrement_ena] -> Switch2/2
  Relational Operator1/1 -> Switch1/2, Logical Operator1/1
  Sum/1 -> Switch1/3, Relational Operator1/1
  DelayTime/1 -> Sum1/1
  Weighted Sample Time/1 -> Sum/2, Sum1/2
  e/1 -> DetectionFront1/1(Entree), Logical Operator/1
  Constant5/1 -> Weighted Sample Time/1
  Logical Operator1/1 -> Logical Operator/2

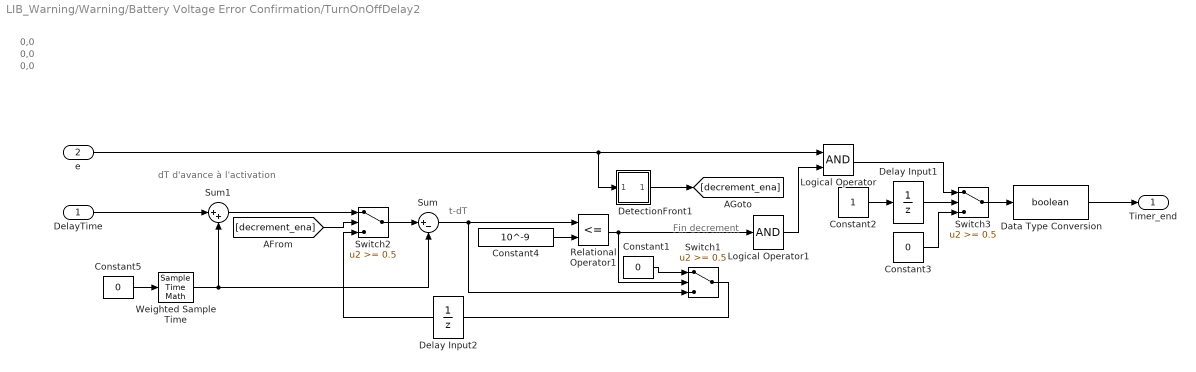
== system LIB_Warning/Warning/Battery Voltage Error Confirmation/TurnOnOffDelay2 ==
  note: dT d'avance à l'activation
  note: t-dT
  note: Fin decrement
  note: 0,0
  note: 0,0
  note: 0,0
  note: 0,0
  note: 0,0
  note: 0,0
  note: 0,0
  DelayTime : Inport
  e : Inport  Port=2
  Constant1 : Constant  Value=0
  Constant2 : Constant
  Constant3 : Constant  Value=0
  Constant4 : Constant  Tag=AM,Constant,0,1,Value;CMP,Value;  Value=10^-9
  Constant5 : Constant  Value=0  SampleTime=-1
  Data Type Conversion : DataTypeConversion  OutDataTypeStr=boolean
  Delay Input1 : UnitDelay  Description=\nStore in Global RAM  SampleTime=-1
  Delay Input2 : UnitDelay  Description=\nStore in Global RAM  SampleTime=-1
  DetectionFront1 : Subsystem  mask(DETECTIONFRONT){FrontType=Rising, InitialValue=0}
      mask prompts: FrontType "Type de front :"; InitialValue "Condition initiale :"
      mask help:
      | Detecte un front sur un signal binaire :
      | - descendant (Falling)
      | - montant (Rising)
      | - les deux (Either).
      mask init:
      | if (FrontType==1);x=[0 1 1 2];y=[0 0 1 1];
      | elseif (FrontType==2);x=[0 1 1 2];y=[1 1 0 0];
      | else;x=[0 1 1 2;3 4 4 5]';y=[0 0 1 1;1 1 0 0]';end;
      mask TypeOptions FrontType: Rising | Falling | Either
      mask Display: plot(x,y)
  Logical Operator : Logic  AllPortsSameDT=off  OutDataTypeStr=boolean
  Logical Operator1 : Logic  Inputs=1  AllPortsSameDT=off  OutDataTypeStr=boolean
  Relational Operator1 : RelationalOperator  Operator=<=  ZeroCross=off  RndMeth=Nearest
  Sum : Sum  Inputs=|+-
  Sum1 : Sum  Inputs=|++
  Switch1 : Switch  Tag=GEN,Threshold;AM,Switch,2,1;CMP,Threshold;  Threshold=0.5  SaturateOnIntegerOverflow=on
  Switch2 : Switch  Tag=GEN,Threshold;AM,Switch,2,1;CMP,Threshold;  Threshold=0.5  SaturateOnIntegerOverflow=on
  Switch3 : Switch  Tag=GEN,Threshold;AM,Switch,2,1;CMP,Threshold;  Threshold=0.5  SaturateOnIntegerOverflow=on
  Weighted Sample Time : SampleTimeMath  TsampMathOp=Ts Only
  Timer_end : Outport
  wires:
  Logical Operator1/1 -> Logical Operator/2
  Constant5/1 -> Weighted Sample Time/1
  e/1 -> Logical Operator/1, DetectionFront1/1(Entree)
  Weighted Sample Time/1 -> Sum1/2, Sum/2
  DelayTime/1 -> Sum1/1
  Sum/1 -> Relational Operator1/1, Switch1/3
  Relational Operator1/1 -> Logical Operator1/1, Switch1/2
  [decrement_ena] -> Switch2/2
  Sum1/1 -> Switch2/1
  Switch2/1 -> Sum/1
  Delay Input2/1 -> Switch2/3
  Constant1/1 -> Switch1/1
  Switch1/1 -> Delay Input2/1
  DetectionFront1/1(Front) -> [decrement_ena]
  Constant4/1 -> Relational Operator1/2
  Constant2/1 -> Delay Input1/1
  Delay Input1/1 -> Switch3/2
  Switch3/1 -> Data Type Conversion/1
  Logical Operator/1 -> Switch3/1
  Constant3/1 -> Switch3/3
  Data Type Conversion/1 -> Timer_end/1

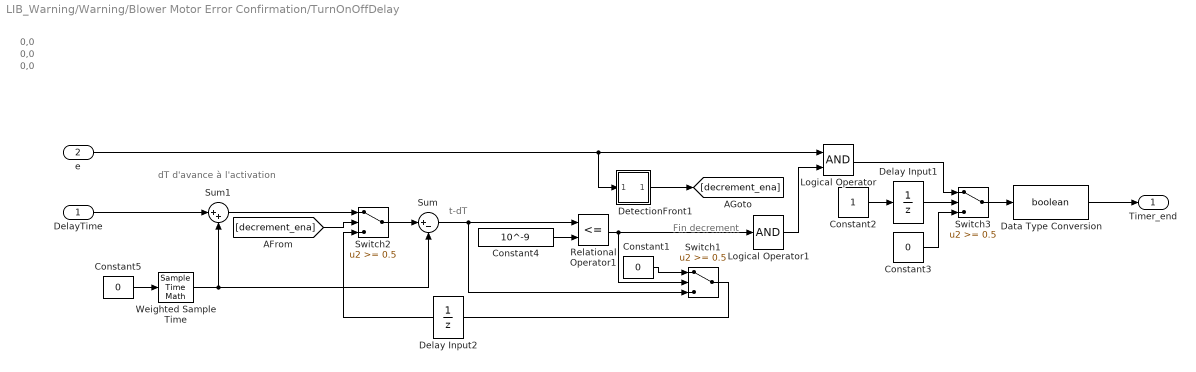
== system LIB_Warning/Warning/Blower Motor Error Confirmation/TurnOnOffDelay ==
  note: 0,0
  note: 0,0
  note: 0,0
  note: 0,0
  note: 0,0
  note: 0,0
  note: 0,0
  note: Fin decrement
  note: t-dT
  note: dT d'avance à l'activation
  DelayTime : Inport
  e : Inport  Port=2
  Constant1 : Constant  Value=0
  Constant2 : Constant
  Constant3 : Constant  Value=0
  Constant4 : Constant  Tag=AM,Constant,0,1,Value;CMP,Value;  Value=10^-9
  Constant5 : Constant  Value=0  SampleTime=-1
  Data Type Conversion : DataTypeConversion  OutDataTypeStr=boolean
  Delay Input1 : UnitDelay  Description=\nStore in Global RAM  SampleTime=-1
  Delay Input2 : UnitDelay  Description=\nStore in Global RAM  SampleTime=-1
  DetectionFront1 : Subsystem  mask(DETECTIONFRONT){FrontType=Rising, InitialValue=0}
      mask prompts: FrontType "Type de front :"; InitialValue "Condition initiale :"
      mask help:
      | Detecte un front sur un signal binaire :
      | - descendant (Falling)
      | - montant (Rising)
      | - les deux (Either).
      mask init:
      | if (FrontType==1);x=[0 1 1 2];y=[0 0 1 1];
      | elseif (FrontType==2);x=[0 1 1 2];y=[1 1 0 0];
      | else;x=[0 1 1 2;3 4 4 5]';y=[0 0 1 1;1 1 0 0]';end;
      mask TypeOptions FrontType: Rising | Falling | Either
      mask Display: plot(x,y)
  Logical Operator : Logic  AllPortsSameDT=off  OutDataTypeStr=boolean
  Logical Operator1 : Logic  Inputs=1  AllPortsSameDT=off  OutDataTypeStr=boolean
  Relational Operator1 : RelationalOperator  Operator=<=  ZeroCross=off  RndMeth=Nearest
  Sum : Sum  Inputs=|+-
  Sum1 : Sum  Inputs=|++
  Switch1 : Switch  Tag=GEN,Threshold;AM,Switch,2,1;CMP,Threshold;  Threshold=0.5  SaturateOnIntegerOverflow=on
  Switch2 : Switch  Tag=GEN,Threshold;AM,Switch,2,1;CMP,Threshold;  Threshold=0.5  SaturateOnIntegerOverflow=on
  Switch3 : Switch  Tag=GEN,Threshold;AM,Switch,2,1;CMP,Threshold;  Threshold=0.5  SaturateOnIntegerOverflow=on
  Weighted Sample Time : SampleTimeMath  TsampMathOp=Ts Only
  Timer_end : Outport
  wires:
  Data Type Conversion/1 -> Timer_end/1
  Constant3/1 -> Switch3/3
  Logical Operator/1 -> Switch3/1
  Switch3/1 -> Data Type Conversion/1
  Delay Input1/1 -> Switch3/2
  Constant2/1 -> Delay Input1/1
  Constant4/1 -> Relational Operator1/2
  DetectionFront1/1(Front) -> [decrement_ena]
  Switch1/1 -> Delay Input2/1
  Constant1/1 -> Switch1/1
  Delay Input2/1 -> Switch2/3
  Switch2/1 -> Sum/1
  Sum1/1 -> Switch2/1
  [decrement_ena] -> Switch2/2
  Relational Operator1/1 -> Switch1/2, Logical Operator1/1
  Sum/1 -> Switch1/3, Relational Operator1/1
  DelayTime/1 -> Sum1/1
  Weighted Sample Time/1 -> Sum/2, Sum1/2
  e/1 -> DetectionFront1/1(Entree), Logical Operator/1
  Constant5/1 -> Weighted Sample Time/1
  Logical Operator1/1 -> Logical Operator/2

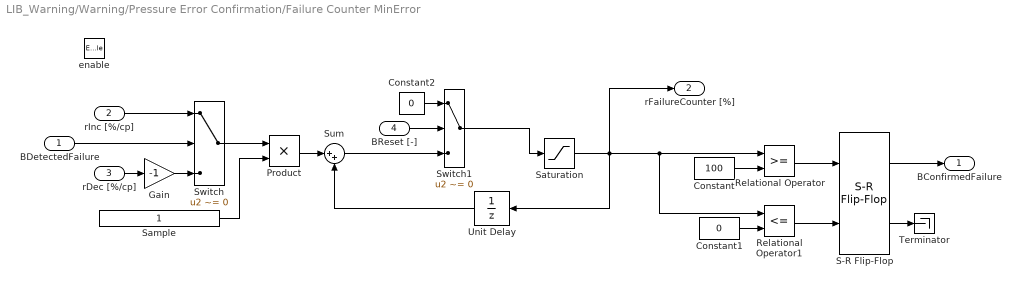
== system LIB_Warning/Warning/Pressure Error Confirmation/Failure Counter MinError ==
  BDetectedFailure : Inport
  rInc [%/cp] : Inport  Port=2
  rDec [%/cp] : Inport  Port=3
  BReset [-] : Inport  Port=4
  enable : EnablePort
  Constant : Constant  Value=100
  Constant1 : Constant  Value=0
  Constant2 : Constant  Value=0
  Gain : Gain  Gain=-1
  Product : Product  RndMeth=Zero
  Relational Operator : RelationalOperator  OutDataTypeStr=boolean  RndMeth=Nearest
  Relational Operator1 : RelationalOperator  Operator=<=  OutDataTypeStr=boolean  RndMeth=Nearest
  S-R Flip-Flop : simulink_extras/Flip Flops/S-R Flip-Flop  initial_condition=0
  Sample : Constant
  Saturation : Saturate  UpperLimit=100  LowerLimit=0
      settings: AttributesFormatString=[%<LowerLimit>;%<UpperLimit>]
  Sum : Sum  Inputs=|++
  Switch : Switch  Criteria=u2 ~= 0
  Switch1 : Switch  Criteria=u2 ~= 0
  Terminator : Terminator
  Unit Delay : UnitDelay  SampleTime=-1
  BConfirmedFailure : Outport
  rFailureCounter [%] : Outport  Port=2
  wires:
  Product/1 -> Sum/1
  Sample/1 -> Product/2
  Gain/1 -> Switch/3
  Constant1/1 -> Relational Operator1/2
  Relational Operator1/1 -> S-R Flip-Flop/2
  Relational Operator/1 -> S-R Flip-Flop/1
  Constant/1 -> Relational Operator/2
  Saturation/1 -> Relational Operator1/1, Relational Operator/1, rFailureCounter [%]/1, Unit Delay/1
  Unit Delay/1 -> Sum/2
  S-R Flip-Flop/1 -> BConfirmedFailure/1
  Sum/1 -> Switch1/3
  Switch/1 -> Product/1
  rDec [%/cp]/1 -> Gain/1
  rInc [%/cp]/1 -> Switch/1
  BDetectedFailure/1 -> Switch/2
  S-R Flip-Flop/2 -> Terminator/1
  Constant2/1 -> Switch1/1
  BReset [-]/1 -> Switch1/2
  Switch1/1 -> Saturation/1

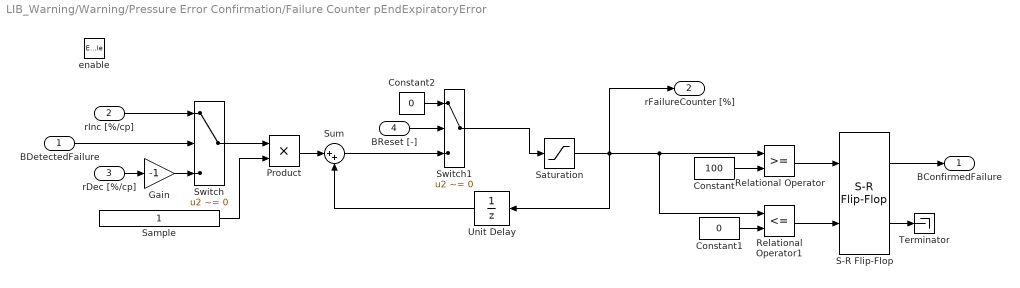
== system LIB_Warning/Warning/Pressure Error Confirmation/Failure Counter pEndExpiratoryError ==
  BDetectedFailure : Inport
  rInc [%/cp] : Inport  Port=2
  rDec [%/cp] : Inport  Port=3
  BReset [-] : Inport  Port=4
  enable : EnablePort
  Constant : Constant  Value=100
  Constant1 : Constant  Value=0
  Constant2 : Constant  Value=0
  Gain : Gain  Gain=-1
  Product : Product  RndMeth=Zero
  Relational Operator : RelationalOperator  OutDataTypeStr=boolean  RndMeth=Nearest
  Relational Operator1 : RelationalOperator  Operator=<=  OutDataTypeStr=boolean  RndMeth=Nearest
  S-R Flip-Flop : simulink_extras/Flip Flops/S-R Flip-Flop  initial_condition=0
  Sample : Constant
  Saturation : Saturate  UpperLimit=100  LowerLimit=0
      settings: AttributesFormatString=[%<LowerLimit>;%<UpperLimit>]
  Sum : Sum  Inputs=|++
  Switch : Switch  Criteria=u2 ~= 0
  Switch1 : Switch  Criteria=u2 ~= 0
  Terminator : Terminator
  Unit Delay : UnitDelay  SampleTime=-1
  BConfirmedFailure : Outport
  rFailureCounter [%] : Outport  Port=2
  wires:
  Product/1 -> Sum/1
  Sample/1 -> Product/2
  Gain/1 -> Switch/3
  Constant1/1 -> Relational Operator1/2
  Relational Operator1/1 -> S-R Flip-Flop/2
  Relational Operator/1 -> S-R Flip-Flop/1
  Constant/1 -> Relational Operator/2
  Saturation/1 -> Relational Operator1/1, Relational Operator/1, rFailureCounter [%]/1, Unit Delay/1
  Unit Delay/1 -> Sum/2
  S-R Flip-Flop/1 -> BConfirmedFailure/1
  Sum/1 -> Switch1/3
  Switch/1 -> Product/1
  rDec [%/cp]/1 -> Gain/1
  rInc [%/cp]/1 -> Switch/1
  BDetectedFailure/1 -> Switch/2
  S-R Flip-Flop/2 -> Terminator/1
  Constant2/1 -> Switch1/1
  BReset [-]/1 -> Switch1/2
  Switch1/1 -> Saturation/1

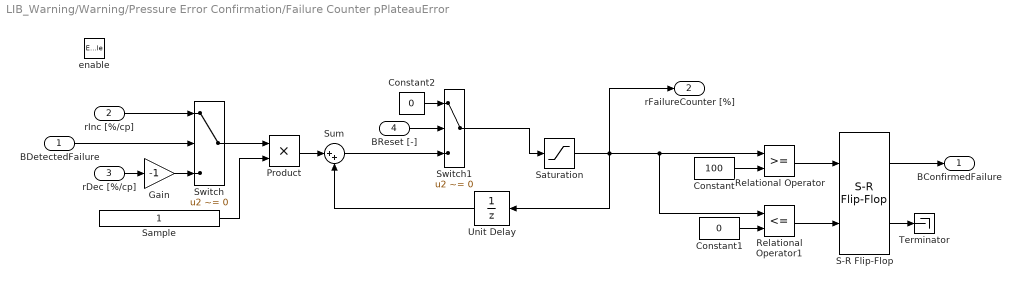
== system LIB_Warning/Warning/Pressure Error Confirmation/Failure Counter pPlateauError ==
  BDetectedFailure : Inport
  rInc [%/cp] : Inport  Port=2
  rDec [%/cp] : Inport  Port=3
  BReset [-] : Inport  Port=4
  enable : EnablePort
  Constant : Constant  Value=100
  Constant1 : Constant  Value=0
  Constant2 : Constant  Value=0
  Gain : Gain  Gain=-1
  Product : Product  RndMeth=Zero
  Relational Operator : RelationalOperator  OutDataTypeStr=boolean  RndMeth=Nearest
  Relational Operator1 : RelationalOperator  Operator=<=  OutDataTypeStr=boolean  RndMeth=Nearest
  S-R Flip-Flop : simulink_extras/Flip Flops/S-R Flip-Flop  initial_condition=0
  Sample : Constant
  Saturation : Saturate  UpperLimit=100  LowerLimit=0
      settings: AttributesFormatString=[%<LowerLimit>;%<UpperLimit>]
  Sum : Sum  Inputs=|++
  Switch : Switch  Criteria=u2 ~= 0
  Switch1 : Switch  Criteria=u2 ~= 0
  Terminator : Terminator
  Unit Delay : UnitDelay  SampleTime=-1
  BConfirmedFailure : Outport
  rFailureCounter [%] : Outport  Port=2
  wires:
  Switch1/1 -> Saturation/1
  BReset [-]/1 -> Switch1/2
  Constant2/1 -> Switch1/1
  S-R Flip-Flop/2 -> Terminator/1
  BDetectedFailure/1 -> Switch/2
  rInc [%/cp]/1 -> Switch/1
  rDec [%/cp]/1 -> Gain/1
  Switch/1 -> Product/1
  Sum/1 -> Switch1/3
  S-R Flip-Flop/1 -> BConfirmedFailure/1
  Unit Delay/1 -> Sum/2
  Saturation/1 -> Unit Delay/1, rFailureCounter [%]/1, Relational Operator/1, Relational Operator1/1
  Constant/1 -> Relational Operator/2
  Relational Operator/1 -> S-R Flip-Flop/1
  Relational Operator1/1 -> S-R Flip-Flop/2
  Constant1/1 -> Relational Operator1/2
  Gain/1 -> Switch/3
  Sample/1 -> Product/2
  Product/1 -> Sum/1

== system LIB_Warning/Warning/Battery Voltage Error Confirmation/TurnOnOffDelay/DetectionFront1 ==
  note: 0,0
  note: 0,0
  note: 0,0
  note: 0,0
  note: 0,0
  note: 0,0
  note: 0,0
  Entree : Inport
  Data Type Conversion : DataTypeConversion  OutDataTypeStr=boolean
  Data Type Conversion1 : DataTypeConversion  OutDataTypeStr=double
  DetectionType : MultiPortSwitch  SaturateOnIntegerOverflow=on  InputSameDT=on
  Either : Logic  Operator=OR
  Falling : RelationalOperator  Operator=<  RndMeth=Nearest  InputSameDT=on
  Memoire2 : Memory  InitialCondition=InitialValue  InheritSampleTime=on
  Rising : RelationalOperator  Operator=>  RndMeth=Nearest  InputSameDT=on
  Sum5 : Sum  Inputs=+-  SaturateOnIntegerOverflow=on  InputSameDT=on  OutDataTypeStr=Inherit: Same as first input
  pedale26 : Constant  Value=1/2
  pedale27 : Constant  Value=-1/2
  pedale28 : Constant  Value=FrontType
  Front : Outport  InitialOutput=0
  wires:
  Data Type Conversion1/1 -> Sum5/1, Memoire2/1
  Data Type Conversion/1 -> Front/1
  pedale28/1 -> DetectionType/1
  Rising/1 -> Either/2, DetectionType/2
  pedale27/1 -> Falling/2
  pedale26/1 -> Rising/2
  Falling/1 -> Either/1, DetectionType/3
  Either/1 -> DetectionType/4
  DetectionType/1 -> Data Type Conversion/1
  Sum5/1 -> Falling/1, Rising/1
  Entree/1 -> Data Type Conversion1/1
  Memoire2/1 -> Sum5/2

== system LIB_Warning/Warning/Battery Voltage Error Confirmation/TurnOnOffDelay1/DetectionFront1 ==
  note: 0,0
  note: 0,0
  note: 0,0
  note: 0,0
  note: 0,0
  note: 0,0
  note: 0,0
  Entree : Inport
  Data Type Conversion : DataTypeConversion  OutDataTypeStr=boolean
  Data Type Conversion1 : DataTypeConversion  OutDataTypeStr=double
  DetectionType : MultiPortSwitch  SaturateOnIntegerOverflow=on  InputSameDT=on
  Either : Logic  Operator=OR
  Falling : RelationalOperator  Operator=<  RndMeth=Nearest  InputSameDT=on
  Memoire2 : Memory  InitialCondition=InitialValue  InheritSampleTime=on
  Rising : RelationalOperator  Operator=>  RndMeth=Nearest  InputSameDT=on
  Sum5 : Sum  Inputs=+-  SaturateOnIntegerOverflow=on  InputSameDT=on  OutDataTypeStr=Inherit: Same as first input
  pedale26 : Constant  Value=1/2
  pedale27 : Constant  Value=-1/2
  pedale28 : Constant  Value=FrontType
  Front : Outport  InitialOutput=0
  wires:
  Memoire2/1 -> Sum5/2
  Entree/1 -> Data Type Conversion1/1
  Sum5/1 -> Rising/1, Falling/1
  DetectionType/1 -> Data Type Conversion/1
  Either/1 -> DetectionType/4
  Falling/1 -> DetectionType/3, Either/1
  pedale26/1 -> Rising/2
  pedale27/1 -> Falling/2
  Rising/1 -> DetectionType/2, Either/2
  pedale28/1 -> DetectionType/1
  Data Type Conversion/1 -> Front/1
  Data Type Conversion1/1 -> Memoire2/1, Sum5/1

== system LIB_Warning/Warning/Battery Voltage Error Confirmation/TurnOnOffDelay2/DetectionFront1 ==
  note: 0,0
  note: 0,0
  note: 0,0
  note: 0,0
  note: 0,0
  note: 0,0
  note: 0,0
  Entree : Inport
  Data Type Conversion : DataTypeConversion  OutDataTypeStr=boolean
  Data Type Conversion1 : DataTypeConversion  OutDataTypeStr=double
  DetectionType : MultiPortSwitch  SaturateOnIntegerOverflow=on  InputSameDT=on
  Either : Logic  Operator=OR
  Falling : RelationalOperator  Operator=<  RndMeth=Nearest  InputSameDT=on
  Memoire2 : Memory  InitialCondition=InitialValue  InheritSampleTime=on
  Rising : RelationalOperator  Operator=>  RndMeth=Nearest  InputSameDT=on
  Sum5 : Sum  Inputs=+-  SaturateOnIntegerOverflow=on  InputSameDT=on  OutDataTypeStr=Inherit: Same as first input
  pedale26 : Constant  Value=1/2
  pedale27 : Constant  Value=-1/2
  pedale28 : Constant  Value=FrontType
  Front : Outport  InitialOutput=0
  wires:
  Data Type Conversion1/1 -> Sum5/1, Memoire2/1
  Data Type Conversion/1 -> Front/1
  pedale28/1 -> DetectionType/1
  Rising/1 -> Either/2, DetectionType/2
  pedale27/1 -> Falling/2
  pedale26/1 -> Rising/2
  Falling/1 -> Either/1, DetectionType/3
  Either/1 -> DetectionType/4
  DetectionType/1 -> Data Type Conversion/1
  Sum5/1 -> Falling/1, Rising/1
  Entree/1 -> Data Type Conversion1/1
  Memoire2/1 -> Sum5/2

== system LIB_Warning/Warning/Blower Motor Error Confirmation/TurnOnOffDelay/DetectionFront1 ==
  note: 0,0
  note: 0,0
  note: 0,0
  note: 0,0
  note: 0,0
  note: 0,0
  note: 0,0
  Entree : Inport
  Data Type Conversion : DataTypeConversion  OutDataTypeStr=boolean
  Data Type Conversion1 : DataTypeConversion  OutDataTypeStr=double
  DetectionType : MultiPortSwitch  SaturateOnIntegerOverflow=on  InputSameDT=on
  Either : Logic  Operator=OR
  Falling : RelationalOperator  Operator=<  RndMeth=Nearest  InputSameDT=on
  Memoire2 : Memory  InitialCondition=InitialValue  InheritSampleTime=on
  Rising : RelationalOperator  Operator=>  RndMeth=Nearest  InputSameDT=on
  Sum5 : Sum  Inputs=+-  SaturateOnIntegerOverflow=on  InputSameDT=on  OutDataTypeStr=Inherit: Same as first input
  pedale26 : Constant  Value=1/2
  pedale27 : Constant  Value=-1/2
  pedale28 : Constant  Value=FrontType
  Front : Outport  InitialOutput=0
  wires:
  Memoire2/1 -> Sum5/2
  Entree/1 -> Data Type Conversion1/1
  Sum5/1 -> Rising/1, Falling/1
  DetectionType/1 -> Data Type Conversion/1
  Either/1 -> DetectionType/4
  Falling/1 -> DetectionType/3, Either/1
  pedale26/1 -> Rising/2
  pedale27/1 -> Falling/2
  Rising/1 -> DetectionType/2, Either/2
  pedale28/1 -> DetectionType/1
  Data Type Conversion/1 -> Front/1
  Data Type Conversion1/1 -> Memoire2/1, Sum5/1
